simulink model "modelMotor1"  (R2015a)
settings: Solver=ode45  StartTime=0.0  StopTime=2  RelTol=1e-3
values from neighbouring files (symbols this model uses):
  J = 8.5e-7    (= 8.5e-07)    [motorModel.m]    (also in relayModel.m = 3.89475e-08)
  KG = 0.0159    [motorModel.m]
  KGT = 1419    [motorModel.m]
  MR = 2.4e-3    (= 0.0024)    [motorModel.m]
  R_Amarture = 4.64    [motorModel.m]
settings Model: Creator=Big Boy  LastModifiedBy=Big Boy

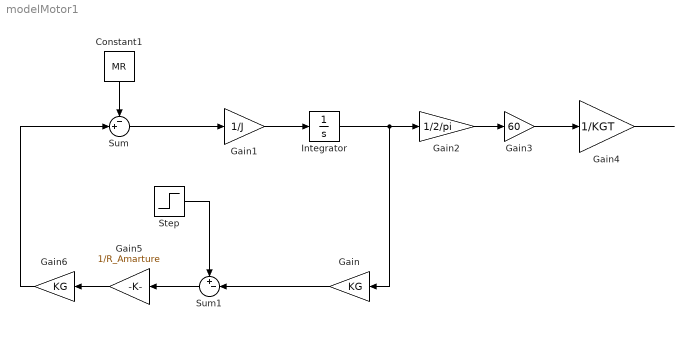
== system modelMotor1 ==
  Constant1 : Constant  Value=MR
  Gain : Gain  Gain=KG
  Gain1 : Gain  Gain=1/J
  Gain2 : Gain  Gain=1/2/pi
  Gain3 : Gain  Gain=60
  Gain4 : Gain  Gain=1/KGT
  Gain5 : Gain  Gain=1/R_Amarture
  Gain6 : Gain  Gain=KG
  Integrator : Integrator
  Step : Step  Time=0  After=5  SampleTime=0
  Sum : Sum  Inputs=-+|
  Sum1 : Sum  Inputs=+-|
  wires:
  Sum1/1 -> Gain5/1
  Gain/1 -> Sum1/2
  Integrator/1 -> Gain/1, Gain2/1
  Gain2/1 -> Gain3/1
  Gain3/1 -> Gain4/1
  Gain4/1 -> ?
  Constant1/1 -> Sum/1
  Sum/1 -> Gain1/1
  Gain1/1 -> Integrator/1
  Gain5/1 -> Gain6/1
  Gain6/1 -> Sum/2
  Step/1 -> Sum1/1
